simulink subsystem "PieroBel_Model"  (R2023b)
settings: Solver=VariableStepAuto  StartTime=0.0  StopTime=10.0  RelTol=1e-3
settings Model: Creator=marqu  LastModifiedBy=marqu

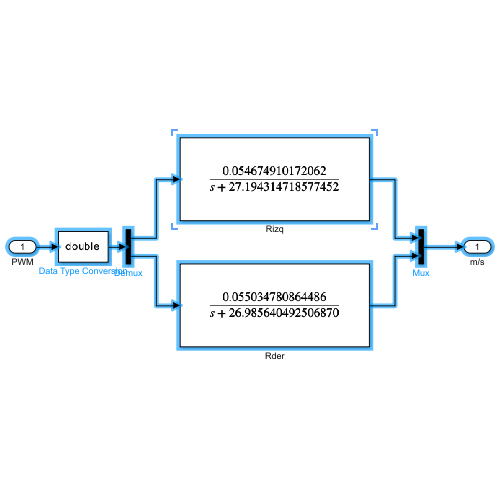
[thumbnail: Simulink's stored preview of the top-level diagram]
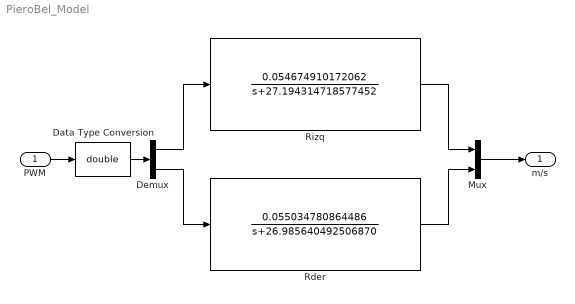
== system PieroBel_Model ==
  PWM : Inport
  Data Type Conversion : DataTypeConversion  OutDataTypeStr=double  SaturateOnIntegerOverflow=off  RndMeth=Floor
  Demux : Demux  Outputs=2
  Mux : Mux  Inputs=2
  Rder : TransferFcn  Numerator=[0.055034780864486]  Denominator=[1,26.985640492506870]
  Rizq : TransferFcn  Numerator=[0.054674910172062]  Denominator=[1,27.194314718577452]
  m/s : Outport
  wires:
  PWM/1 -> Data Type Conversion/1
  Data Type Conversion/1 -> Demux/1
  Rder/1 -> Mux/2
  Rizq/1 -> Mux/1
  Mux/1 -> m/s/1
  Demux/2 -> Rder/1
  Demux/1 -> Rizq/1
